simulink model "one_leaderfollow_formationcontrol"  (R2019a)
settings: Solver=ode23  StartTime=0.0  StopTime=30  RelTol=1e-3
undefined symbols (not defined in the file): B, I, L
settings Model: Creator=DELL  LastModifiedBy=DELL

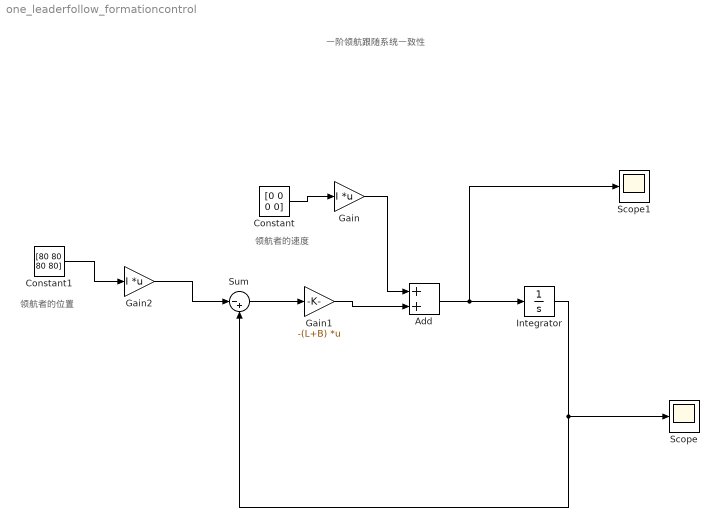
== system one_leaderfollow_formationcontrol ==
  note: 一阶领航跟随系统一致性
  note: 领航者的速度
  note: 领航者的位置
  Add : Sum
  Constant : Constant  Value=[0 0 0 0]
  Constant1 : Constant  Value=[80 80 80 80]
  Gain : Gain  Gain=I  Multiplication=Matrix(K*u)
  Gain1 : Gain  Gain=-(L+B)  Multiplication=Matrix(K*u)
  Gain2 : Gain  Gain=I  Multiplication=Matrix(K*u)
  Integrator : Integrator  InitialCondition=[20 10 40 0]
  Scope : Scope
  Scope1 : Scope
  Sum : Sum  Inputs=|-+
  wires:
  Constant/1 -> Gain/1
  Gain/1 -> Add/1
  Add/1 -> Scope1/1, Integrator/1
  Gain1/1 -> Add/2
  Sum/1 -> Gain1/1
  Integrator/1 -> Scope/1, Sum/2
  Constant1/1 -> Gain2/1
  Gain2/1 -> Sum/1
